simulink model "SIM_DNNs"  (R2024a)
settings: Solver=VariableStepAuto  StartTime=0.0  StopTime=xs.sim.Tf2  FixedStep=1e-4  RelTol=1e-3
values from neighbouring files (symbols this model uses):
  eval_net_func1 = Simulink.Parameter    [InitMain.m]    (also in InitMain_original.m)
  eval_net_func2 = Simulink.Parameter    [InitMain.m]    (also in InitMain_original.m)
  mins_max1 = Simulink.Parameter    [InitMain.m]    (also in InitMain_original.m)
  mins_max2 = Simulink.Parameter    [InitMain.m]    (also in InitMain_original.m)
  parsDNN1 = Simulink.Parameter    [InitMain.m]    (also in InitMain_original.m)
  parsDNN2 = Simulink.Parameter    [InitMain.m]    (also in InitMain_original.m)
  use_net1 = Simulink.Parameter    [InitMain.m]    (also in InitMain_original.m)
  use_net2 = Simulink.Parameter    [InitMain.m]    (also in InitMain_original.m)
  xmpc1 = xs.MPC1    [InitMPCs.m]
  xmpc2 = xs.MPC2    [InitMPCs.m]
  xproj1 = xs.Proj1    [InitMPCs.m]
  xs = xs_us(1:4)    [MPC1_f.m]    (also in MPC2_f.m = xs_us(1:3))
undefined symbols (not defined in the file or in its folder): Lf, Rf, xsat2
libraries: spsThreePhaseSeriesRLCBranchLib x4, spsThreePhaseVIMeasurementLib x3, spsTriangleGeneratorLib x2, spsDCVoltageSourceLib x1, spsThreePhaseBreakerLib x1, spsThreePhaseSourceLib x1, spsTwoLevelConverterLib x1, sps_lib x1
settings Model: Creator=iaaco  LastModifiedBy=fabus
settings SolverCC: ShapePreserveControl=EnableAll
settings OptimizationCC: DefaultParameterBehavior=Inlined  EnhancedBackFolding=on  PassReuseOutputArgsAs=Individual arguments  ZeroExternalMemoryAtStartup=off  ZeroInternalMemoryAtStartup=off  OptimizeBlockOrder=speed  DifferentSizesBufferReuse=on  OptimizationCustomize=off  EfficientTunableParamExpr=on
settings DebuggingCC: ParameterTunabilityLossMsg=error
settings RTWCC: Description=Embedded Coder  SystemTargetFile=ert.tlc  TemplateMakefile=ert_default_tmf
settings CodeAppCC: ForceParamTrailComments=on  IgnoreCustomStorageClasses=off  OperatorAnnotations=on  SimulinkDataObjDesc=on  SFDataObjDesc=on  InsertBlockDesc=on
settings ERTTargetCC: TargetLangStandard=C99 (ISO)  GenerateSampleERTMain=on  InlinedParameterPlacement=NonHierarchical  ERTCustomFileTemplate=example_file_process.tlc

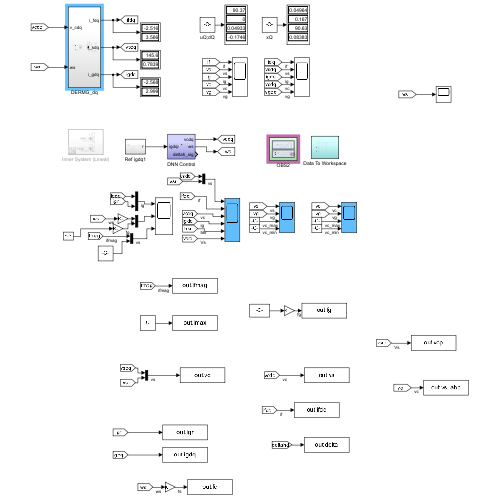
[thumbnail: Simulink's stored preview of the top-level diagram]
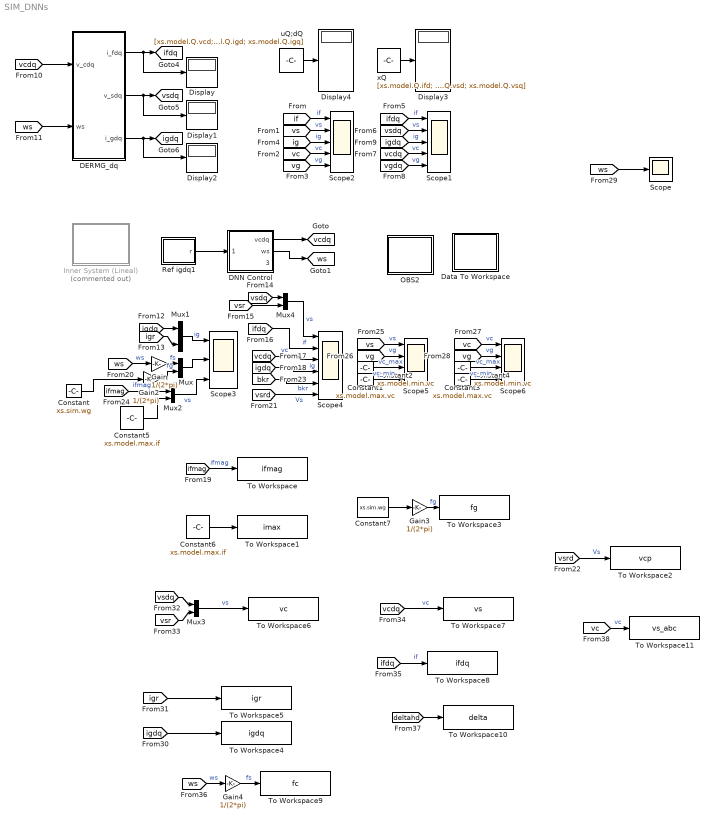
== system SIM_DNNs ==
  Constant : Constant  Value=xs.sim.wg
  Constant1 : Constant  Value=xs.model.max.vc
  Constant2 : Constant  Value=xs.model.min.vc
  Constant3 : Constant  Value=xs.model.max.vc
  Constant4 : Constant  Value=xs.model.min.vc
  Constant5 : Constant  Value=xs.model.max.if
  Constant6 : Constant  Value=xs.model.max.if
  Constant7 : Constant  Value=xs.sim.wg
  DERMG_dq : Subsystem
  DNN Control : Subsystem
  Data To Workspace : Subsystem
  Display{,1..4} (5 alike) : Display
  Gain{,2..4} (4 alike) : Gain  Gain=1/(2*pi)
  Inner System (Lineal) : Subsystem  Commented=on
  Mux{,1..4} (5 alike) : Mux  Inputs=2
  OBS2 : Subsystem
  Ref igdq1 : Subsystem
  Scope : Scope
  Scope1 : Scope  NumInputPorts=5
  Scope2 : Scope  NumInputPorts=5
  Scope3 : Scope  NumInputPorts=3
  Scope4 : Scope  NumInputPorts=6
  Scope5 : Scope  NumInputPorts=4
  Scope6 : Scope  NumInputPorts=4
  To Workspace : ToWorkspace  VariableName=ifmag  SampleTime=-1
  To Workspace1 : ToWorkspace  VariableName=imax  SampleTime=-1
  To Workspace10 : ToWorkspace  VariableName=delta  SaveFormat=Timeseries  SampleTime=-1
  To Workspace11 : ToWorkspace  VariableName=vs_abc  SaveFormat=Timeseries  SampleTime=-1
  To Workspace2 : ToWorkspace  VariableName=vcp  SaveFormat=Timeseries  SampleTime=-1
  To Workspace3 : ToWorkspace  VariableName=fg  SampleTime=-1
  To Workspace4 : ToWorkspace  VariableName=igdq  SaveFormat=Timeseries  SampleTime=-1
  To Workspace5 : ToWorkspace  VariableName=igr  SaveFormat=Timeseries  SampleTime=-1
  To Workspace6 : ToWorkspace  VariableName=vc  SaveFormat=Timeseries  SampleTime=-1
  To Workspace7 : ToWorkspace  VariableName=vs  SaveFormat=Timeseries  SampleTime=-1
  To Workspace8 : ToWorkspace  VariableName=ifdq  SaveFormat=Timeseries  SampleTime=-1
  To Workspace9 : ToWorkspace  VariableName=fc  SaveFormat=Timeseries  SampleTime=-1
  uQ;dQ : Constant  Value=[xs.model.Q.vcd; xs.model.Q.vcq; xs.model.Q.igd; xs.model.Q.igq]
  xQ : Constant  Value=[xs.model.Q.ifd; xs.model.Q.ifq; xs.model.Q.vsd; xs.model.Q.vsq]
  tag scope: ifdq=global, igdq=global, vcdq=global, vsdq=global, ws=global
  wires:
  [vcdq] -> Scope1/4  "vc"
  [ifdq] -> Scope1/1  "if"
  [vgdq] -> Scope1/5  "vg"
  [igdq] -> Scope1/3  "ig"
  [vsdq] -> Scope1/2  "vs"
  [vcdq] -> DERMG_dq/1(v_cdq)
  [ws] -> DERMG_dq/2(ws)
  DERMG_dq/1(i_fdq) -> Display/1, [ifdq]
  DERMG_dq/2(v_sdq) -> Display1/1, [vsdq]
  DERMG_dq/3(i_gdq) -> Display2/1, [igdq]
  xQ/1 -> Display3/1
  uQ;dQ/1 -> Display4/1
  Ref igdq1/1(r) -> DNN Control/1(igdqr)
  DNN Control/1(vcdq) -> [vcdq]
  DNN Control/2(ws) -> [ws]
  [ig] -> Scope2/3  "ig"
  [vs] -> Scope2/2  "vs"
  [vg] -> Scope2/5  "vg"
  [if] -> Scope2/1  "if"
  [vc] -> Scope2/4  "vc"
  Constant4/1 -> Scope6/4  "vc_min"
  Gain2/1 -> Mux/2  "fg"
  Constant3/1 -> Scope6/3  "vc_max"
  [vc] -> Scope6/1  "vc"
  [vg] -> Scope5/2  "vg"
  [igr] -> Mux1/2
  Gain/1 -> Mux/1  "fs"
  Mux/1 -> Scope3/2
  [vcdq] -> Scope4/3  "vc"
  [bkr] -> Scope4/5  "bkr"
  [vg] -> Scope6/2  "vg"
  [vs] -> Scope5/1  "vs"
  [igdq] -> Mux1/1
  Constant1/1 -> Scope5/3  "vc_max"
  Constant/1 -> Gain2/1
  Constant2/1 -> Scope5/4  "vc_min"
  [igdq] -> Scope4/4  "ig"
  [vsdq] -> Mux4/1
  Mux4/1 -> Scope4/1  "vs"
  [vsrd] -> Scope4/6  "Vs"
  [ws] -> Gain/1  "ws"
  [vsr] -> Mux4/2
  Mux1/1 -> Scope3/1  "ig"
  [ws] -> Scope/1
  [ifdq] -> Scope4/2  "if"
  Constant5/1 -> Mux2/2
  [ifmag] -> Mux2/1  "ifmag"
  Mux2/1 -> Scope3/3  "vs"
  [ifmag] -> To Workspace/1  "ifmag"
  Constant6/1 -> To Workspace1/1
  Constant7/1 -> Gain3/1
  Gain3/1 -> To Workspace3/1  "fg"
  [igdq] -> To Workspace4/1
  [igr] -> To Workspace5/1
  Mux3/1 -> To Workspace6/1  "vs"
  [vsr] -> Mux3/2
  [vsdq] -> Mux3/1
  [vcdq] -> To Workspace7/1  "vc"
  [ifdq] -> To Workspace8/1  "if"
  [ws] -> Gain4/1  "ws"
  Gain4/1 -> To Workspace9/1  "fs"
  [vsrd] -> To Workspace2/1  "Vs"
  [deltahd] -> To Workspace10/1
  [vc] -> To Workspace11/1  "vc"

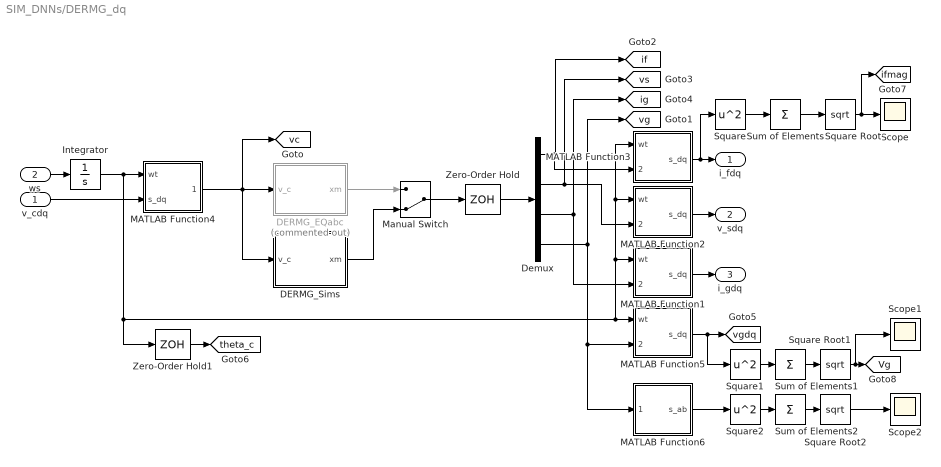
== system SIM_DNNs/DERMG_dq ==
  v_cdq : Inport
  ws : Inport  Port=2
  DERMG_EQabc : Subsystem  Commented=on
  DERMG_Sims : Subsystem
  Demux : Demux
  Integrator : Integrator  WrapState=on
  MATLAB Function1 : MATLAB Function  TreatAsAtomicUnit=on
  MATLAB Function2 : MATLAB Function  TreatAsAtomicUnit=on
  MATLAB Function3 : MATLAB Function  TreatAsAtomicUnit=on
  MATLAB Function4 : MATLAB Function  TreatAsAtomicUnit=on
  MATLAB Function5 : MATLAB Function  TreatAsAtomicUnit=on
  MATLAB Function6 : MATLAB Function  TreatAsAtomicUnit=on
  Manual Switch : ManualSwitch  CurrentSetting=0
  Scope : Scope
  Scope1 : Scope
  Scope2 : Scope
  Square : Math  Operator=square
  Square Root : Sqrt
  Square Root1 : Sqrt
  Square Root2 : Sqrt
  Square1 : Math  Operator=square
  Square2 : Math  Operator=square
  Sum of Elements : Sum  Inputs=+
  Sum of Elements1 : Sum  Inputs=+
  Sum of Elements2 : Sum  Inputs=+
  Zero-Order Hold : ZeroOrderHold  SampleTime=xs.model.Ts
  Zero-Order Hold1 : ZeroOrderHold  SampleTime=xs.model.Ts
  i_fdq : Outport
  v_sdq : Outport  Port=2
  i_gdq : Outport  Port=3
  tag scope: Vg=global, if=global, ifmag=global, ig=global, theta_c=global, vc=global, vg=global, vgdq=global, vs=global
  wires:
  MATLAB Function3/1(s_dq) -> Square/1, i_fdq/1
  MATLAB Function2/1(s_dq) -> v_sdq/1
  MATLAB Function1/1(s_dq) -> i_gdq/1
  ws/1 -> Integrator/1
  Square/1 -> Sum of Elements/1
  Sum of Elements/1 -> Square Root/1
  Integrator/1 -> MATLAB Function5/1(wt), MATLAB Function1/1(wt), MATLAB Function3/1(wt), MATLAB Function2/1(wt), Zero-Order Hold1/1, MATLAB Function4/1(wt)
  Demux/1 -> MATLAB Function3/2(s_abc), [if]
  Demux/2 -> MATLAB Function2/2(s_abc), [vs]
  Demux/3 -> MATLAB Function1/2(s_abc), [ig]
  Demux/4 -> MATLAB Function6/1(s_abc), MATLAB Function5/2(s_abc), [vg]
  Square Root/1 -> [ifmag], Scope/1
  Zero-Order Hold/1 -> Demux/1
  Zero-Order Hold1/1 -> [theta_c]
  MATLAB Function4/1(s_abc) -> [vc], DERMG_Sims/1(v_c), DERMG_EQabc/1(v_c)
  Manual Switch/1 -> Zero-Order Hold/1
  DERMG_EQabc/1(xm) -> Manual Switch/1
  DERMG_Sims/1(xm) -> Manual Switch/2
  Sum of Elements1/1 -> Square Root1/1
  MATLAB Function5/1(s_dq) -> Square1/1, [vgdq]
  Square1/1 -> Sum of Elements1/1
  Square Root1/1 -> Scope1/1, [Vg]
  Square Root2/1 -> Scope2/1
  Square2/1 -> Sum of Elements2/1
  Sum of Elements2/1 -> Square Root2/1
  MATLAB Function6/1(s_ab) -> Square2/1
  v_cdq/1 -> MATLAB Function4/2(s_dq)

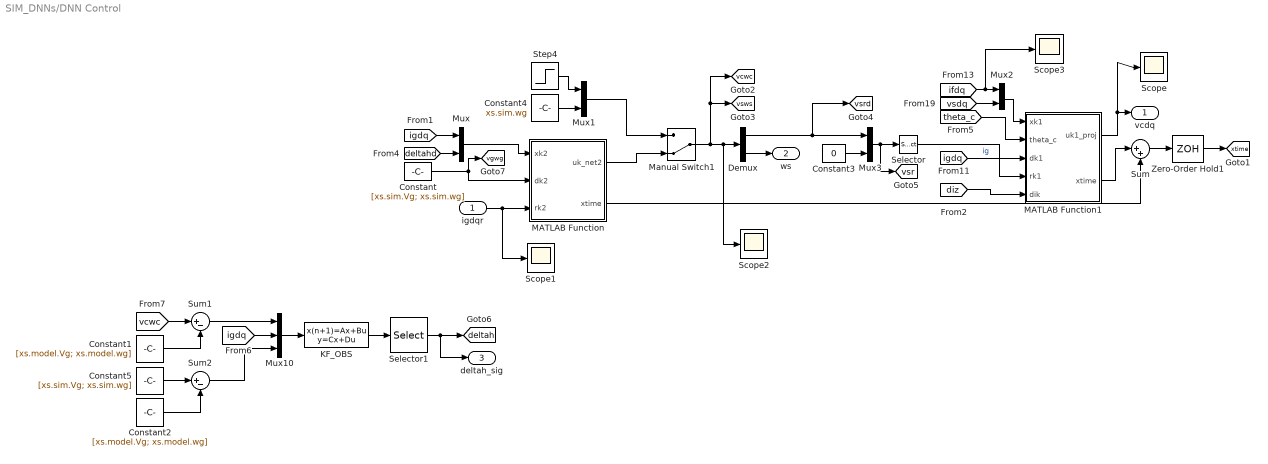
== system SIM_DNNs/DNN Control ==
  igdqr : Inport
  Constant : Constant  Value=[xs.sim.Vg; xs.sim.wg]
  Constant1 : Constant  Value=[xs.model.Vg; xs.model.wg]
  Constant2 : Constant  Value=[xs.model.Vg; xs.model.wg]
  Constant3 : Constant  Value=0
  Constant4 : Constant  Value=xs.sim.wg
  Constant5 : Constant  Value=[xs.sim.Vg; xs.sim.wg]
  Demux : Demux  Outputs=2
  KF_OBS : DiscreteStateSpace  A=xs.model.Ad2-xs.OBS2.L*xs.model.C2s  B=[xs.model.Bd2 ,xs.OBS2.L,xs.model.Bod2]  C=eye(3)  D=zeros(3,6)  InitialCondition=zeros(3,1)  SampleTime=xs.model.Ts
  MATLAB Function : MATLAB Function  TreatAsAtomicUnit=on  SystemSampleTime=xs.model.Ts
  MATLAB Function1 : MATLAB Function  TreatAsAtomicUnit=on  SystemSampleTime=xs.model.Ts
  Manual Switch1 : ManualSwitch  CurrentSetting=0
  Mux{,1..3} (4 alike) : Mux  Inputs=2
  Mux10 : Mux  Inputs=3
  Scope{,1..3} (4 alike) : Scope
  Selector : Selector  InputPortWidth=2  IndexOptions=Index vector (dialog)  Indices=[1]  OutputSizes=1
  Selector1 : Selector  InputPortWidth=3  IndexOptions=Index vector (dialog)  Indices=[3]  OutputSizes=1
  Step4 : Step  Time=xs.sim.vsdr.Tstep  Before=90  After=xs.sim.vsdr.XF  SampleTime=0
  Sum : Sum  Inputs=|++
  Sum1 : Sum  Inputs=|+-
  Sum2 : Sum  Inputs=|+-
  Zero-Order Hold1 : ZeroOrderHold  SampleTime=xs.model.Ts
  vcdq : Outport
  ws : Outport  Port=2
  deltah_sig : Outport  Port=3
  tag scope: deltah=global, vcwc=global, vgwg=global, vsr=global, vsrd=global, vsws=global, xtime=global
  wires:
  Manual Switch1/1 -> [vcwc], [vsws], Scope2/1, Demux/1
  Mux1/1 -> Manual Switch1/1
  [deltahd] -> Mux/2
  Constant/1 -> [vgwg], MATLAB Function/2(dk2)
  [igdq] -> Mux/1
  Mux/1 -> MATLAB Function/1(xk2)
  igdqr/1 -> Scope1/1, MATLAB Function/3(rk2)
  MATLAB Function/1(uk_net2) -> Manual Switch1/2
  [ifdq] -> Scope3/1, Mux2/1
  Constant3/1 -> Mux3/2
  [vsdq] -> Mux2/2
  Mux3/1 -> Selector/1, [vsr]
  Demux/1 -> Mux3/1, [vsrd]
  Mux2/1 -> MATLAB Function1/1(xk1)
  Demux/2 -> ws/1
  [theta_c] -> MATLAB Function1/2(theta_c)
  Constant4/1 -> Mux1/2
  Step4/1 -> Mux1/1
  MATLAB Function1/1(uk1_proj) -> Scope/1, vcdq/1
  MATLAB Function1/2(xtime) -> Sum/1
  MATLAB Function/2(xtime) -> Sum/2
  Sum/1 -> Zero-Order Hold1/1
  Zero-Order Hold1/1 -> [xtime]
  Selector/1 -> MATLAB Function1/4(rk1)
  [igdq] -> MATLAB Function1/3(dk1)  "ig"
  [diz] -> MATLAB Function1/5(dik)
  Mux10/1 -> KF_OBS/1
  Sum1/1 -> Mux10/1
  [vcwc] -> Sum1/1
  [igdq] -> Mux10/2
  Constant5/1 -> Sum2/1
  KF_OBS/1 -> Selector1/1
  Constant1/1 -> Sum1/2
  Sum2/1 -> Mux10/3
  Selector1/1 -> deltah_sig/1, [deltah]
  Constant2/1 -> Sum2/2

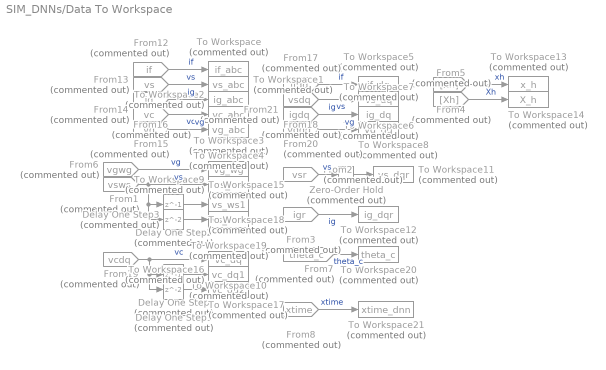
== system SIM_DNNs/Data To Workspace ==
  Delay One Step : Delay  Commented=on  DelayLength=1  SampleTime=xs.model.Ts
  Delay One Step1 : Delay  Commented=on  SampleTime=xs.model.Ts
  Delay One Step2 : Delay  Commented=on  DelayLength=1  SampleTime=xs.model.Ts
  Delay One Step3 : Delay  Commented=on  SampleTime=xs.model.Ts
  From1 : From  Commented=on  GotoTag=vsws  TagVisibility=global
  From12 : From  Commented=on  GotoTag=if  TagVisibility=global
  From13 : From  Commented=on  GotoTag=vs  TagVisibility=global
  From14 : From  Commented=on  GotoTag=vc  TagVisibility=global
  From15 : From  Commented=on  GotoTag=vg  TagVisibility=global
  From16 : From  Commented=on  GotoTag=ig  TagVisibility=global
  From17 : From  Commented=on  GotoTag=ifdq  TagVisibility=global
  From18 : From  Commented=on  GotoTag=vsdq  TagVisibility=global
  From19 : From  Commented=on  GotoTag=vcdq  TagVisibility=global
  From2 : From  Commented=on  GotoTag=vsr  TagVisibility=global
  From20 : From  Commented=on  GotoTag=vgdq  TagVisibility=global
  From21 : From  Commented=on  GotoTag=igdq  TagVisibility=global
  From3 : From  Commented=on  GotoTag=igr  TagVisibility=global
  From4 : From  Commented=on  GotoTag=xh
  From5 : From  Commented=on  GotoTag=Xh
  From6 : From  Commented=on  GotoTag=vgwg  TagVisibility=global
  From7 : From  Commented=on  GotoTag=theta_c  TagVisibility=global
  From8 : From  Commented=on  GotoTag=xtime  TagVisibility=global
  To Workspace : ToWorkspace  Commented=on  VariableName=if_abc  SaveFormat=Structure With Time  SampleTime=xs.model.Ts
  To Workspace1 : ToWorkspace  Commented=on  VariableName=vs_abc  SaveFormat=Structure With Time  SampleTime=xs.model.Ts
  To Workspace10 : ToWorkspace  Commented=on  VariableName=vc_dq  SaveFormat=Structure With Time  SampleTime=xs.model.Ts
  To Workspace11 : ToWorkspace  Commented=on  VariableName=vs_dqr  SaveFormat=Structure With Time  SampleTime=xs.model.Ts
  To Workspace12 : ToWorkspace  Commented=on  VariableName=ig_dqr  SaveFormat=Structure With Time  SampleTime=xs.model.Ts
  To Workspace13 : ToWorkspace  Commented=on  VariableName=x_h  SaveFormat=Structure With Time  SampleTime=xs.model.Ts
  To Workspace14 : ToWorkspace  Commented=on  VariableName=X_h  SaveFormat=Structure With Time  SampleTime=xs.model.Ts
  To Workspace15 : ToWorkspace  Commented=on  VariableName=vg_wg  SaveFormat=Structure With Time  SampleTime=xs.model.Ts
  To Workspace16 : ToWorkspace  Commented=on  VariableName=vc_dq1  SaveFormat=Structure With Time  SampleTime=xs.model.Ts
  To Workspace17 : ToWorkspace  Commented=on  VariableName=vc_dq2  SaveFormat=Structure With Time  SampleTime=xs.model.Ts
  To Workspace18 : ToWorkspace  Commented=on  VariableName=vs_ws1  SaveFormat=Structure With Time  SampleTime=xs.model.Ts
  To Workspace19 : ToWorkspace  Commented=on  VariableName=vs_ws2  SaveFormat=Structure With Time  SampleTime=xs.model.Ts
  To Workspace2 : ToWorkspace  Commented=on  VariableName=ig_abc  SaveFormat=Structure With Time  SampleTime=xs.model.Ts
  To Workspace20 : ToWorkspace  Commented=on  VariableName=theta_c  SaveFormat=Structure With Time  SampleTime=xs.model.Ts
  To Workspace21 : ToWorkspace  Commented=on  VariableName=xtime_dnn  SaveFormat=Structure With Time  SampleTime=xs.model.Ts
  To Workspace3 : ToWorkspace  Commented=on  VariableName=vc_abc  SaveFormat=Structure With Time  SampleTime=xs.model.Ts
  To Workspace4 : ToWorkspace  Commented=on  VariableName=vg_abc  SaveFormat=Structure With Time  SampleTime=xs.model.Ts
  To Workspace5 : ToWorkspace  Commented=on  VariableName=if_dq  SaveFormat=Structure With Time  SampleTime=xs.model.Ts
  To Workspace6 : ToWorkspace  Commented=on  VariableName=vs_dq  SaveFormat=Structure With Time  SampleTime=xs.model.Ts
  To Workspace7 : ToWorkspace  Commented=on  VariableName=ig_dq  SaveFormat=Structure With Time  SampleTime=xs.model.Ts
  To Workspace8 : ToWorkspace  Commented=on  VariableName=vg_dq  SaveFormat=Structure With Time  SampleTime=xs.model.Ts
  To Workspace9 : ToWorkspace  Commented=on  VariableName=vs_ws  SaveFormat=Structure With Time  SampleTime=xs.model.Ts
  Zero-Order Hold : ZeroOrderHold  Commented=on  SampleTime=xs.model.Ts
  wires:
  From12/1 -> To Workspace/1  "if"
  From13/1 -> To Workspace1/1  "vs"
  From16/1 -> To Workspace2/1  "ig"
  From14/1 -> To Workspace3/1  "vc"
  From15/1 -> To Workspace4/1  "vg"
  From17/1 -> To Workspace5/1  "if"
  From18/1 -> To Workspace6/1  "vs"
  From21/1 -> To Workspace7/1  "ig"
  From20/1 -> To Workspace8/1  "vg"
  From1/1 -> Delay One Step3/1, Delay One Step2/1, To Workspace9/1  "vs"
  From19/1 -> Delay One Step1/1, Delay One Step/1, To Workspace10/1  "vc"
  From3/1 -> To Workspace12/1  "ig"
  Zero-Order Hold/1 -> To Workspace11/1
  From4/1 -> To Workspace13/1  "xh"
  From5/1 -> To Workspace14/1  "Xh"
  From6/1 -> To Workspace15/1  "vg"
  From2/1 -> Zero-Order Hold/1  "vs"
  Delay One Step/1 -> To Workspace16/1
  Delay One Step1/1 -> To Workspace17/1
  Delay One Step2/1 -> To Workspace18/1
  Delay One Step3/1 -> To Workspace19/1
  From7/1 -> To Workspace20/1  "theta_c"
  From8/1 -> To Workspace21/1  "xtime"

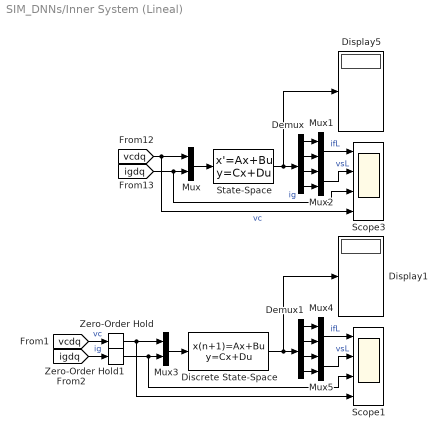
== system SIM_DNNs/Inner System (Lineal) ==
  Demux : Demux
  Demux1 : Demux
  Discrete State-Space : DiscreteStateSpace  A=xs.model.Ad1  B=[xs.model.Bd1,xs.model.Bod1]  C=eye(4)  D=zeros(4)  InitialCondition=[xs.model.Q.ifd ; xs.model.Q.ifq ; xs.model.Q.vsd ; xs.model.Q.vsq]  SampleTime=xs.model.Ts
  Display1 : Display
  Display5 : Display
  Mux{,1..5} (6 alike) : Mux  Inputs=2
  Scope1 : Scope  NumInputPorts=4
  Scope3 : Scope  NumInputPorts=4
  State-Space : StateSpace  A=xs.model.A1  B=[xs.model.B1,xs.model.Bo1]  C=eye(4)  D=zeros(4)  InitialCondition=[xs.model.Q.ifd ; xs.model.Q.ifq ; xs.model.Q.vsd ; xs.model.Q.vsq]
  Zero-Order Hold : ZeroOrderHold  SampleTime=xs.model.Ts
  Zero-Order Hold1 : ZeroOrderHold  SampleTime=xs.model.Ts
  wires:
  Mux/1 -> State-Space/1
  Demux/1 -> Mux1/1
  Demux/2 -> Mux1/2
  State-Space/1 -> Display5/1, Demux/1
  [vcdq] -> Scope3/4, Mux/1  "vc"
  [igdq] -> Scope3/3, Mux/2  "ig"
  Mux2/1 -> Scope3/2  "vsL"
  Mux1/1 -> Scope3/1  "ifL"
  Demux/3 -> Mux2/1
  Demux/4 -> Mux2/2
  Demux1/4 -> Mux5/2
  [vcdq] -> Zero-Order Hold/1  "vc"
  Mux5/1 -> Scope1/2  "vsL"
  Demux1/2 -> Mux4/2
  Mux3/1 -> Discrete State-Space/1
  [igdq] -> Zero-Order Hold1/1  "ig"
  Demux1/1 -> Mux4/1
  Mux4/1 -> Scope1/1  "ifL"
  Demux1/3 -> Mux5/1
  Discrete State-Space/1 -> Display1/1, Demux1/1
  Zero-Order Hold/1 -> Scope1/4, Mux3/1
  Zero-Order Hold1/1 -> Scope1/3, Mux3/2

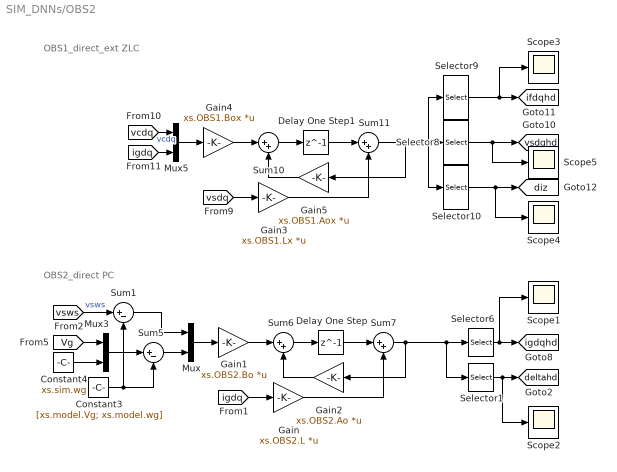
== system SIM_DNNs/OBS2 ==
  note: OBS1_direct_ext ZLC
  note: OBS2_direct PC
  Constant3 : Constant  Value=[xs.model.Vg; xs.model.wg]
  Constant4 : Constant  Value=xs.sim.wg
  Delay One Step : Delay  DelayLength=1  InitialCondition=zeros(3,1)  SampleTime=xs.model.Ts
  Delay One Step1 : Delay  DelayLength=1  InitialCondition=zeros(6,1)  SampleTime=xs.model.Ts
  Gain : Gain  Gain=xs.OBS2.L  Multiplication=Matrix(K*u)
  Gain1 : Gain  Gain=xs.OBS2.Bo  Multiplication=Matrix(K*u)
  Gain2 : Gain  Gain=xs.OBS2.Ao  Multiplication=Matrix(K*u)
  Gain3 : Gain  Gain=xs.OBS1.Lx  Multiplication=Matrix(K*u)
  Gain4 : Gain  Gain=xs.OBS1.Box  Multiplication=Matrix(K*u)
  Gain5 : Gain  Gain=xs.OBS1.Aox  Multiplication=Matrix(K*u)
  Mux : Mux  Inputs=2
  Mux3 : Mux  Inputs=2
  Mux5 : Mux  Inputs=2
  Scope{1..5} (5 alike) : Scope
  Selector1 : Selector  InputPortWidth=3  IndexOptions=Index vector (dialog)  Indices=[3]  OutputSizes=1
  Selector10 : Selector  InputPortWidth=6  IndexOptions=Index vector (dialog)  Indices=[5 6]  OutputSizes=1
  Selector6 : Selector  InputPortWidth=3  IndexOptions=Index vector (dialog)  Indices=[1 2]  OutputSizes=1
  Selector8 : Selector  InputPortWidth=6  IndexOptions=Index vector (dialog)  Indices=[3 4]  OutputSizes=1
  Selector9 : Selector  InputPortWidth=6  IndexOptions=Index vector (dialog)  Indices=[1 2]  OutputSizes=1
  Sum1 : Sum  Inputs=|+-
  Sum{6..7,10..11} (4 alike) : Sum  Inputs=|++
  Sum5 : Sum  Inputs=|+-
  tag scope: deltahd=global, diz=global, ifdqhd=global, igdqhd=global, vsdqhd=global
  wires:
  Sum11/1 -> Selector9/1, Selector10/1, Selector8/1, Gain5/1
  Gain4/1 -> Sum10/1
  [vsdq] -> Gain3/1
  [vsws] -> Sum1/1  "vsws"
  [vcdq] -> Mux5/1  "vcdq"
  Gain1/1 -> Sum6/1
  Gain2/1 -> Sum6/2
  [igdq] -> Gain/1
  Mux/1 -> Gain1/1
  Sum7/1 -> Selector1/1, Selector6/1, Gain2/1
  [igdq] -> Mux5/2
  Selector6/1 -> Scope1/1, [igdqhd]
  Sum6/1 -> Delay One Step/1
  Sum1/1 -> Mux/1
  Sum5/1 -> Mux/2
  Constant4/1 -> Mux3/2
  Mux3/1 -> Sum5/1
  Selector1/1 -> Scope2/1, [deltahd]
  [Vg] -> Mux3/1
  Constant3/1 -> Sum5/2, Sum1/2
  Selector9/1 -> [ifdqhd], Scope3/1
  Gain3/1 -> Sum11/2
  Delay One Step1/1 -> Sum11/1
  Selector8/1 -> Scope5/1, [vsdqhd]
  Mux5/1 -> Gain4/1
  Selector10/1 -> Scope4/1, [diz]
  Delay One Step/1 -> Sum7/1
  Gain/1 -> Sum7/2
  Gain5/1 -> Sum10/2
  Sum10/1 -> Delay One Step1/1

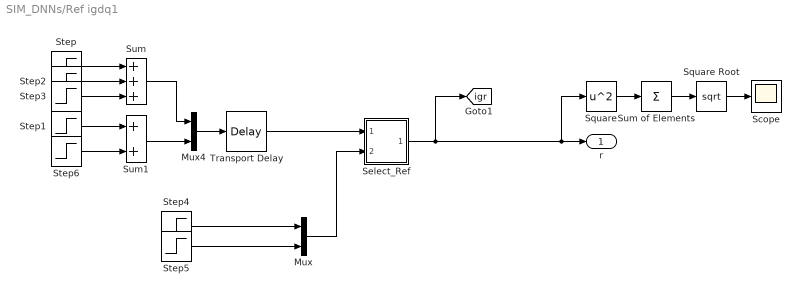
== system SIM_DNNs/Ref igdq1 ==
  Mux : Mux  Inputs=2
  Mux4 : Mux  Inputs=2
  Scope : Scope
  Select_Ref : Subsystem
  Square : Math  Operator=square
  Square Root : Sqrt
  Step : Step  Time=xs.sim.Tf2*0.25  Before=3  After=7  SampleTime=0
  Step1 : Step  Time=xs.sim.Tf2*0.5  After=-7  SampleTime=0
  Step2 : Step  Time=xs.sim.Tf2*0.5  After=-7  SampleTime=0
  Step3 : Step  Time=xs.sim.Tf2*0.75  After=-3  SampleTime=0
  Step4 : Step  Time=xs.sim.igdr.Tstep  Before=xs.sim.igdr.X0  After=xs.sim.igdr.XF  SampleTime=0
  Step5 : Step  Time=xs.sim.igqr.Tstep  Before=xs.sim.igqr.X0  After=xs.sim.igqr.XF  SampleTime=0
  Step6 : Step  Time=xs.sim.Tf2*0.75  After=10  SampleTime=0
  Sum : Sum  Inputs=+++
  Sum of Elements : Sum  Inputs=+
  Sum1 : Sum
  Transport Delay : TransportDelay  DelayTime=0.1  BufferSize=23000
  r : Outport
  tag scope: igr=global
  wires:
  Step4/1 -> Mux/1
  Step5/1 -> Mux/2
  Square Root/1 -> Scope/1
  Square/1 -> Sum of Elements/1
  Select_Ref/1(r2k) -> r/1, Square/1, [igr]
  Sum of Elements/1 -> Square Root/1
  Mux/1 -> Select_Ref/2(In2)
  Transport Delay/1 -> Select_Ref/1(In1)
  Step6/1 -> Sum1/2
  Step3/1 -> Sum/3
  Mux4/1 -> Transport Delay/1
  Step2/1 -> Sum/2
  Step/1 -> Sum/1
  Step1/1 -> Sum1/1
  Sum1/1 -> Mux4/2
  Sum/1 -> Mux4/1

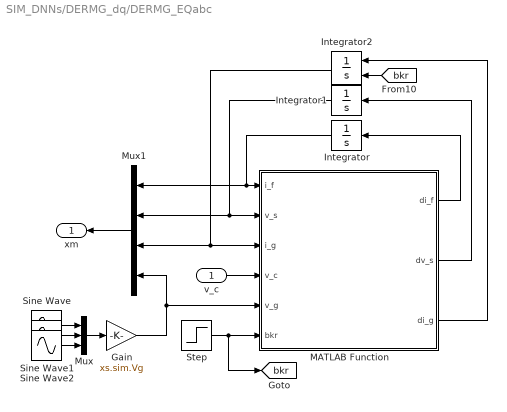
== system SIM_DNNs/DERMG_dq/DERMG_EQabc ==
  v_c : Inport
  Gain : Gain  Gain=xs.sim.Vg
  Integrator : Integrator  InitialCondition=xs.sim.X0abc.if*0
  Integrator1 : Integrator  InitialCondition=xs.sim.X0abc.vs*0
  Integrator2 : Integrator  ExternalReset=falling  InitialCondition=xs.sim.X0abc.ig*0
  MATLAB Function : MATLAB Function  TreatAsAtomicUnit=on
  Mux : Mux  Inputs=3
  Mux1 : Mux
  Sine Wave : Sin  Frequency=xs.sim.wg  Phase=0 + pi/2- xs.sim.thetag0  SampleTime=0
  Sine Wave1 : Sin  Frequency=xs.sim.wg  Phase=-2*pi/3 + pi/2 - xs.sim.thetag0  SampleTime=0
  Sine Wave2 : Sin  Frequency=xs.sim.wg  Phase=-4*pi/3 + pi/2 - xs.sim.thetag0  SampleTime=0
  Step : Step  Time=xs.sim.bkr.Tstep  Before=xs.sim.bkr.X0  After=xs.sim.bkr.XF  SampleTime=0
  xm : Outport
  tag scope: bkr=global
  wires:
  Integrator/1 -> MATLAB Function/1(i_f), Mux1/1
  MATLAB Function/3(di_g) -> Integrator2/1
  Integrator2/1 -> Mux1/3, MATLAB Function/3(i_g)
  MATLAB Function/2(dv_s) -> Integrator1/1
  Integrator1/1 -> Mux1/2, MATLAB Function/2(v_s)
  v_c/1 -> MATLAB Function/4(v_c)
  MATLAB Function/1(di_f) -> Integrator/1
  Sine Wave/1 -> Mux/1
  Mux/1 -> Gain/1
  Sine Wave2/1 -> Mux/3
  Sine Wave1/1 -> Mux/2
  Gain/1 -> MATLAB Function/5(v_g), Mux1/4
  Mux1/1 -> xm/1
  Step/1 -> [bkr], MATLAB Function/6(bkr)
  [bkr] -> Integrator2/2

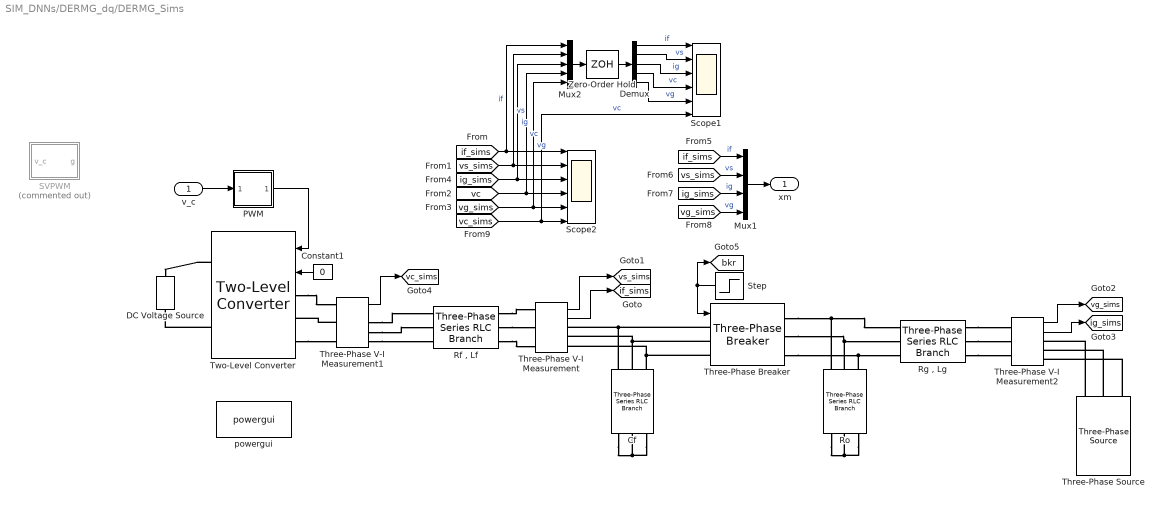
== system SIM_DNNs/DERMG_dq/DERMG_Sims ==
  v_c : Inport
  Cf : spsThreePhaseSeriesRLCBranchLib/Three-Phase Series RLC Branch  LConnTagsString=A|B|C  RConnTagsString=A|B|C  BranchType=C  Resistance=Rf  Inductance=Lf  Capacitance=xs.sim.Cf  Measurements=None
  Constant1 : Constant  Value=0
  DC Voltage Source : spsDCVoltageSourceLib/DC Voltage Source  Amplitude=xs.sim.vdc  Measurements=None
  Demux : Demux  Outputs=5
  Mux1 : Mux
  Mux2 : Mux  Inputs=5
  PWM : Subsystem
  "Rf , Lf" : spsThreePhaseSeriesRLCBranchLib/Three-Phase Series RLC Branch  LConnTagsString=A|B|C  RConnTagsString=A|B|C  BranchType=RL  Resistance=xs.sim.Rf  Inductance=xs.sim.Lf  Capacitance=0  Measurements=None
  "Rg , Lg" : spsThreePhaseSeriesRLCBranchLib/Three-Phase Series RLC Branch  LConnTagsString=A|B|C  RConnTagsString=A|B|C  BranchType=RL  Resistance=xs.sim.Rg  Inductance=xs.sim.Lg  Capacitance=0  Measurements=None
  Ro : spsThreePhaseSeriesRLCBranchLib/Three-Phase Series RLC Branch  LConnTagsString=A|B|C  RConnTagsString=A|B|C  BranchType=R  Resistance=xs.sim.Ro  Inductance=Lf  Capacitance=xs.sim.Cf  Measurements=None
  SVPWM : Subsystem  Commented=on
  Scope1 : Scope  NumInputPorts=6
  Scope2 : Scope  NumInputPorts=6
  Step : Step  Time=xs.sim.bkr.Tstep  Before=xs.sim.bkr.X0  After=xs.sim.bkr.XF  SampleTime=0
  Three-Phase V-I Measurement : spsThreePhaseVIMeasurementLib/Three-Phase V-I Measurement  VoltageMeasurement=phase-to-ground  SetLabelV=off  LabelV=Vabc  Vpu=off  VpuLL=off  CurrentMeasurement=yes  SetLabelI=off  LabelI=Iabc  Ipu=off  Pbase=100e6  Vbase=500e3  OutputType=Complex  PhasorSimulation=off  PSBequivalent=0
  Three-Phase V-I Measurement1 : spsThreePhaseVIMeasurementLib/Three-Phase V-I Measurement  VoltageMeasurement=phase-to-ground  SetLabelV=off  LabelV=Vabc  Vpu=off  VpuLL=off  CurrentMeasurement=yes  SetLabelI=off  LabelI=Iabc  Ipu=off  Pbase=100e6  Vbase=500e3  OutputType=Complex  PhasorSimulation=off  PSBequivalent=0
  Three-Phase V-I Measurement2 : spsThreePhaseVIMeasurementLib/Three-Phase V-I Measurement  VoltageMeasurement=phase-to-ground  SetLabelV=off  LabelV=Vabc  Vpu=off  VpuLL=off  CurrentMeasurement=yes  SetLabelI=off  LabelI=Iabc  Ipu=off  Pbase=100e6  Vbase=500e3  OutputType=Complex  PhasorSimulation=off  PSBequivalent=0
  Three-Phase Breaker : spsThreePhaseBreakerLib/Three-Phase Breaker  InitialState=closed  SwitchA=on  SwitchB=on  SwitchC=on  SwitchTimes="[1/60  5/60]"  External=on  BreakerResistance=0  SnubberResistance=1e4  SnubberCapacitance=inf  Measurements=None
  Three-Phase Source : spsThreePhaseSourceLib/Three-Phase Source  InternalConnection=Yg  VoltagePhases=off  Voltage=xs.sim.Vg*sqrt(3/2)  PhaseAngle=90  Voltage_phases=[25e3 25e3 25e3]/sqrt(3)  PhaseAngles_phases=[0 -120 +120]  Frequency=xs.sim.wg/(2*pi)  NonIdealSource=off  SpecifyImpedance=off  Resistance=0.8929  Inductance=16.58e-3  ShortCircuitLevel=100e6  BaseVoltage=25e3  XRratio=7  BusType=swing  Pref=10e3  Qref=0  Prefabc=[10e3, 10e3, 10e3]  Qrefabc=[0, 0, 0]  Qmin=-inf  Qmax=inf
  Two-Level Converter : spsTwoLevelConverterLib/Two-Level Converter  ModelType=Switching devices  Ron=1e-4  Rs=1e6  Cs=inf  Vforward=[0,0]  Ron_Diode=1e-2  Rs_Diode=1e4  Cs_Diode=inf  Vf_Diode=0  Rs_CurrentSource=inf  Ron_ACsource=1e-5
      settings: LibrarySourceBlock=sps_lib/Power Electronics/Two-Level Converter
  Zero-Order Hold : ZeroOrderHold  SampleTime=xs.model.Ts
  powergui : sps_lib/powergui  Priority=1  SimulationMode=Continuous  SampleTime=xs.model.Ts/5  frequency=60  Iterations=50  frequencyindice=0  Pbase=100e6  ErrMax=1e-4  UnitsV=kV  UnitsW=MW  buscounter=0  FunctionMessages=off  echomessages=off  EnableUseOfTLC=off  CurrentSourceSwitches=off  DisableSnubberDevices=off  DisableRonSwitches=off  DisableVfSwitches=off  DisplayEquations=off  AutomaticDiscreteSolvers=off  SolverType=Tustin/Backward Euler (TBE)  Interpol=off  ExternalGateDelay=off  methode=off  Ts=100  x0status=blocks  SPID=on  SwTol=0  HookPort=off  NonlinearTolerance=1e-4  nMaxIteration=100  ContinueOnMaxIteration=off  RestoreLinks=warning  ResistiveCurrentMeasurement=off  Frange=[0:2:500]  Ylog=off  Xlog=on  ShowGrid=off  save=off  variable=ZData  structure=0  ZoomFFT=off  StartTime=0.0  cycles=1  DisplayStyle=1  fundamental=60  FreqAxis=off  MaxFrequency=1000  frequencyindicesteady=1  RmsSteady=1  display=off
  xm : Outport
  tag scope: bkr=global, if_sims=global, ig_sims=global, vc_sims=global, vg_sims=global, vs_sims=global
  wires:
  Constant1/1 -> Two-Level Converter/2
  [vg_sims] -> Mux2/5, Scope2/5  "vg"
  [ig_sims] -> Mux2/3, Scope2/3  "ig"
  [if_sims] -> Mux2/1, Scope2/1  "if"
  [vs_sims] -> Mux2/2, Scope2/2  "vs"
  [vc] -> Mux2/4, Scope2/4  "vc"
  Three-Phase V-I Measurement/2 -> [if_sims]
  Three-Phase V-I Measurement2/1 -> [vg_sims]
  Three-Phase V-I Measurement2/2 -> [ig_sims]
  [if_sims] -> Mux1/1  "if"
  [vs_sims] -> Mux1/2  "vs"
  [ig_sims] -> Mux1/3  "ig"
  [vg_sims] -> Mux1/4  "vg"
  Three-Phase V-I Measurement/1 -> [vs_sims]
  Mux1/1 -> xm/1
  Three-Phase V-I Measurement1/1 -> [vc_sims]
  [vc_sims] -> Scope1/6, Scope2/6  "vc"
  Mux2/1 -> Zero-Order Hold/1
  Zero-Order Hold/1 -> Demux/1
  Demux/1 -> Scope1/1  "if"
  Demux/2 -> Scope1/2  "vs"
  Demux/3 -> Scope1/3  "ig"
  Demux/4 -> Scope1/4  "vc"
  Demux/5 -> Scope1/5  "vg"
  v_c/1 -> PWM/1(In1)
  PWM/1(Out1) -> Two-Level Converter/1
  Step/1 -> [bkr], Three-Phase Breaker/1
  connections:
  Two-Level Converter/RConn1 -- DC Voltage Source/RConn1
  Two-Level Converter/RConn2 -- DC Voltage Source/LConn1
  "Rf , Lf"/RConn1 -- Three-Phase V-I Measurement/LConn1
  "Rf , Lf"/RConn2 -- Three-Phase V-I Measurement/LConn2
  "Rf , Lf"/RConn3 -- Three-Phase V-I Measurement/LConn3
  Cf/LConn1 -- Three-Phase Breaker/LConn1 -- Three-Phase V-I Measurement/RConn1
  Cf/LConn2 -- Three-Phase V-I Measurement/RConn2 -- Three-Phase Breaker/LConn2
  Cf/LConn3 -- Three-Phase V-I Measurement/RConn3 -- Three-Phase Breaker/LConn3
  Three-Phase Source/RConn1 -- Three-Phase V-I Measurement2/RConn1
  Three-Phase Source/RConn2 -- Three-Phase V-I Measurement2/RConn2
  Three-Phase Source/RConn3 -- Three-Phase V-I Measurement2/RConn3
  Cf/RConn1 -- Cf/RConn2 -- Cf/RConn3
  Three-Phase V-I Measurement1/LConn2 -- Two-Level Converter/LConn2
  Two-Level Converter/LConn1 -- Three-Phase V-I Measurement1/LConn1
  Two-Level Converter/LConn3 -- Three-Phase V-I Measurement1/LConn3
  Three-Phase V-I Measurement1/RConn3 -- "Rf , Lf"/LConn3
  Three-Phase V-I Measurement1/RConn2 -- "Rf , Lf"/LConn2
  Three-Phase V-I Measurement1/RConn1 -- "Rf , Lf"/LConn1
  "Rg , Lg"/RConn1 -- Three-Phase V-I Measurement2/LConn1
  "Rg , Lg"/RConn2 -- Three-Phase V-I Measurement2/LConn2
  "Rg , Lg"/RConn3 -- Three-Phase V-I Measurement2/LConn3
  Three-Phase Breaker/RConn1 -- Ro/LConn1 -- "Rg , Lg"/LConn1
  Three-Phase Breaker/RConn2 -- Ro/LConn2 -- "Rg , Lg"/LConn2
  Three-Phase Breaker/RConn3 -- Ro/LConn3 -- "Rg , Lg"/LConn3
  Ro/RConn3 -- Ro/RConn1 -- Ro/RConn2

== system SIM_DNNs/Ref igdq1/Select_Ref ==
  In1 : Inport
  In2 : Inport  Port=2
  Product : Product
  Product1 : Product
  Ref_Rand : Constant  Value=1 - xs.sim.Ref_Rand
  Ref_Rand_neg : Constant  Value=xs.sim.Ref_Rand
  Sum1 : Sum  Inputs=|++
  r2k : Outport
  wires:
  Product1/1 -> Sum1/2
  Ref_Rand/1 -> Product/2
  In2/1 -> Product1/2
  Product/1 -> Sum1/1
  Ref_Rand_neg/1 -> Product1/1
  Sum1/1 -> r2k/1
  In1/1 -> Product/1

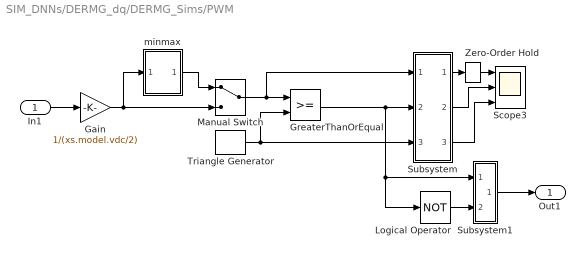
== system SIM_DNNs/DERMG_dq/DERMG_Sims/PWM ==
  In1 : Inport
  Gain : Gain  Gain=1/(xs.model.vdc/2)
  GreaterThanOrEqual : RelationalOperator  OutDataTypeStr=boolean  RndMeth=Simplest  InputSameDT=off
  Logical Operator : Logic  Operator=NOT  AllPortsSameDT=off  OutDataTypeStr=boolean
  Manual Switch : ManualSwitch
  Scope3 : Scope  NumInputPorts=3
  Subsystem : Subsystem
  Subsystem1 : Subsystem
  Triangle Generator : spsTriangleGeneratorLib/Triangle Generator  Freq=1/xs.model.Ts  Phase=0  Ts=0
  Zero-Order Hold : ZeroOrderHold  SampleTime=xs.model.Ts
  minmax : Subsystem
  Out1 : Outport
  wires:
  Triangle Generator/1 -> GreaterThanOrEqual/2, Subsystem/3(In3)
  In1/1 -> Gain/1
  Subsystem/2(Out2) -> Scope3/2
  Subsystem/3(Out3) -> Scope3/3
  GreaterThanOrEqual/1 -> Subsystem/2(In2), Subsystem1/1(In1), Logical Operator/1
  Logical Operator/1 -> Subsystem1/2(In2)
  Subsystem1/1(Out1) -> Out1/1
  Manual Switch/1 -> Subsystem/1(In1), GreaterThanOrEqual/1
  Gain/1 -> minmax/1(In1), Manual Switch/2
  minmax/1(Out1) -> Manual Switch/1
  Subsystem/1(Out1) -> Zero-Order Hold/1
  Zero-Order Hold/1 -> Scope3/1

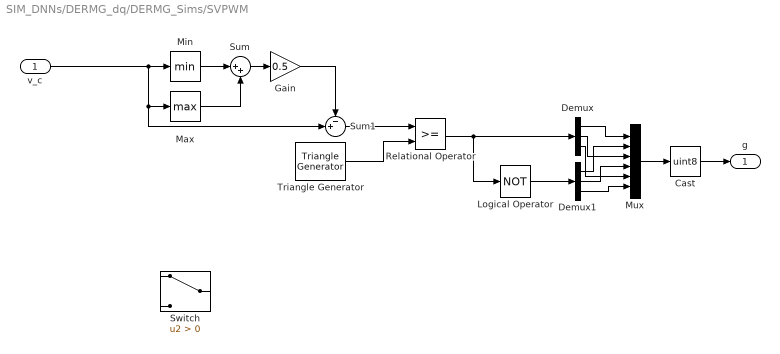
== system SIM_DNNs/DERMG_dq/DERMG_Sims/SVPWM ==
  v_c : Inport
  Cast : DataTypeConversion  OutDataTypeStr=uint8  SaturateOnIntegerOverflow=off  RndMeth=Floor
  Demux : Demux  Outputs=3
  Demux1 : Demux  Outputs=3
  Gain : Gain  Gain=0.5
  Logical Operator : Logic  Operator=NOT  AllPortsSameDT=off  OutDataTypeStr=boolean
  Max : MinMax  Function=max
  Min : MinMax
  Mux : Mux  Inputs=6
  Relational Operator : RelationalOperator  OutDataTypeStr=boolean  ZeroCross=off  RndMeth=Simplest  InputSameDT=off
  Sum : Sum  Inputs=|++
  Sum1 : Sum  Inputs=-+|
  Switch : Switch  Criteria=u2 > Threshold  SaturateOnIntegerOverflow=off  InputSameDT=off
  Triangle Generator : spsTriangleGeneratorLib/Triangle Generator  Freq=2/xs.model.Ts  Phase=0  Ts=0
  g : Outport
  wires:
  v_c/1 -> Max/1, Sum1/2, Min/1
  Sum1/1 -> Relational Operator/1
  Min/1 -> Sum/1
  Triangle Generator/1 -> Relational Operator/2
  Mux/1 -> Cast/1
  Max/1 -> Sum/2
  Demux/1 -> Mux/1
  Logical Operator/1 -> Demux1/1
  Sum/1 -> Gain/1
  Demux1/1 -> Mux/2
  Demux1/2 -> Mux/4
  Demux/3 -> Mux/5
  Relational Operator/1 -> Logical Operator/1, Demux/1
  Demux/2 -> Mux/3
  Demux1/3 -> Mux/6
  Cast/1 -> g/1
  Gain/1 -> Sum1/1

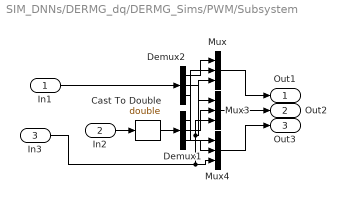
== system SIM_DNNs/DERMG_dq/DERMG_Sims/PWM/Subsystem ==
  In1 : Inport
  In2 : Inport  Port=2
  In3 : Inport  Port=3
  Cast To Double : DataTypeConversion  OutDataTypeStr=double  SaturateOnIntegerOverflow=off  RndMeth=Floor
  Demux1 : Demux  Outputs=3
  Demux2 : Demux  Outputs=3
  Mux : Mux  Inputs=3
  Mux3 : Mux  Inputs=3
  Mux4 : Mux  Inputs=3
  Out1 : Outport
  Out2 : Outport  Port=2
  Out3 : Outport  Port=3
  wires:
  Demux2/2 -> Mux3/1
  In2/1 -> Cast To Double/1
  In3/1 -> Mux3/3, Mux/3, Mux4/3
  Cast To Double/1 -> Demux1/1
  Demux2/3 -> Mux4/1
  Demux1/1 -> Mux/2
  Demux1/3 -> Mux4/2
  Demux2/1 -> Mux/1
  Demux1/2 -> Mux3/2
  Mux/1 -> Out1/1
  Mux3/1 -> Out2/1
  Mux4/1 -> Out3/1
  In1/1 -> Demux2/1

== system SIM_DNNs/DERMG_dq/DERMG_Sims/PWM/Subsystem1 ==
  In1 : Inport
  In2 : Inport  Port=2
  Cast To Double1 : DataTypeConversion  OutDataTypeStr=double  SaturateOnIntegerOverflow=off  RndMeth=Floor
  Demux3 : Demux  Outputs=3
  Demux4 : Demux  Outputs=3
  Mux5 : Mux  Inputs=6
  Out1 : Outport
  wires:
  Mux5/1 -> Cast To Double1/1
  Demux3/3 -> Mux5/5
  Demux3/2 -> Mux5/3
  Demux4/1 -> Mux5/2
  Demux4/2 -> Mux5/4
  Demux3/1 -> Mux5/1
  Demux4/3 -> Mux5/6
  In2/1 -> Demux4/1
  Cast To Double1/1 -> Out1/1
  In1/1 -> Demux3/1

== system SIM_DNNs/DERMG_dq/DERMG_Sims/PWM/minmax ==
  In1 : Inport
  Gain1 : Gain  Gain=0.5
  Max : MinMax  Function=max
  Min : MinMax
  Sum : Sum  Inputs=|++
  Sum1 : Sum  Inputs=-+|
  Out1 : Outport
  wires:
  In1/1 -> Max/1, Min/1, Sum1/2
  Sum/1 -> Gain1/1
  Gain1/1 -> Sum1/1
  Max/1 -> Sum/2
  Min/1 -> Sum/1
  Sum1/1 -> Out1/1

== matlab function SIM_DNNs/DERMG_dq/MATLAB Function2 ==
  data: wt input; s_dq output size=2; s_abc input size=3
function s_dq = abc2dq(wt,s_abc)

% ABC to DQ0 transformation
% s_abc = [a;b;c]
% s_dq0 = [d;q;0]

% Clarke transformation matrix, depends on the electrical angle
T = (2/3)*[cos(wt) cos(wt-2*pi/3) cos(wt+2*pi/3);...
    -sin(wt) -sin(wt-2*pi/3) -sin(wt+2*pi/3);...
    0.5 0.5 0.5];

% DQ0 transformation (only D and Q components are needed)
s_dq0 = T*s_abc;
s_dq = s_dq0(1:2);

end

== matlab function SIM_DNNs/DERMG_dq/MATLAB Function3 ==
  data: wt input; s_dq output size=2; s_abc input size=3
function s_dq = abc2dq(wt,s_abc)

% ABC to DQ0 transformation
% s_abc = [a;b;c]
% s_dq0 = [d;q;0]

% Clarke transformation matrix, depends on the electrical angle
T = (2/3)*[cos(wt) cos(wt-2*pi/3) cos(wt+2*pi/3);...
    -sin(wt) -sin(wt-2*pi/3) -sin(wt+2*pi/3);...
    0.5 0.5 0.5];

% DQ0 transformation (only D and Q components are needed)
s_dq0 = T*s_abc;
s_dq = s_dq0(1:2);

end

== matlab function SIM_DNNs/DERMG_dq/MATLAB Function4 ==
  data: wt input; s_abc output; s_dq input
function s_abc = dq2abc(wt,s_dq)

% DQ0 to ABC transformation
% s_dq0 = [d;q;0]
% s_abc = [a;b;c]

% Inverse Clarke transformation matrix, depends on the electrical angle
Tinv = [cos(wt) -sin(wt) 1;...
    cos(wt-2*pi/3) -sin(wt-2*pi/3) 1;...
    cos(wt+2*pi/3) -sin(wt+2*pi/3) 1];

s_dq0 = [s_dq;0];
s_abc = Tinv*s_dq0;

end

== matlab function SIM_DNNs/DNN Control/MATLAB Function1 ==
  data: xk1 input size=4; theta_c input size=1; uk1_proj output size=2; dk1 input size=2; rk1 input size=1; dik input size=2; xproj1 parameter; xtime output size=1; parsDNN1 parameter; mins_max1 parameter; eval_net_func1 parameter; xmpc1 parameter; use_net1 parameter
function [uk1_proj, xtime] = DNN1(xk1, theta_c, dk1, rk1, dik,xproj1, parsDNN1, mins_max1, eval_net_func1, xmpc1, use_net1)

tStart = tic;
persistent F_
if(use_net1)
    X1 = [xk1; dk1; rk1; cos(theta_c); sin(theta_c)];
    if isempty(F_)
        F_ = fimath('OverflowAction', 'Saturate', ... 
           'RoundingMethod', 'Convergent', ...
           'ProductMode', 'SpecifyPrecision', ...
           'ProductWordLength', parsDNN1.wordLength, ...
           'ProductFractionLength', parsDNN1.fracLength, ...
           'SumMode', 'SpecifyPrecision', ...
           'SumWordLength', parsDNN1.wordLength, ...
           'SumFractionLength', parsDNN1.fracLength);
    end
    %Normalizar
    x_norm = (X1 - mins_max1.in_min) ./ (mins_max1.in_max - mins_max1.in_min);
    %Evaluar
    eval_net_func_char = char(eval_net_func1);
    uk_net1 = double(zeros(size(mins_max1.out_max)));
    uk_net1 = feval(eval_net_func_char,x_norm, parsDNN1, F_);
    %Desnormalizar
    uk_net1 = (mins_max1.out_max - mins_max1.out_min).*uk_net1 + mins_max1.out_min;
    % Output Saturation/Projection
    %uk1_proj = uk_net1 - dik;
    uk1_proj = Project1_f(xk1, uk_net1 - dik, dk1, theta_c, xproj1);
    %uk1_proj= uk_net1;
    % %uk1_proj = min(max(uk1_proj, mins_max1.out_min), mins_max1.out_max);
else
    uk1_proj = MPC1_f(xk1,dk1,[rk1;0],dik,theta_c,xmpc1);
end
xtime = toc(tStart);

end

== matlab function SIM_DNNs/DERMG_dq/DERMG_EQabc/MATLAB Function ==
  data: i_f input; di_f output; v_s input; i_g input; v_c input; v_g input; bkr input; dv_s output; di_g output; xs parameter
function [di_f,dv_s,di_g] = DERMG_SYSEQabc(i_f,v_s,i_g,v_c,v_g,bkr,xs)


[di_f,dv_s,di_g] = DERMG_SYSEQabc_f(i_f,v_s,i_g,v_c,v_g,bkr,xs);


end

== matlab function SIM_DNNs/DERMG_dq/MATLAB Function1 ==
  data: wt input; s_dq output size=2; s_abc input size=3
function s_dq = abc2dq(wt,s_abc)

% ABC to DQ0 transformation
% s_abc = [a;b;c]
% s_dq0 = [d;q;0]

% Clarke transformation matrix, depends on the electrical angle
T = (2/3)*[cos(wt) cos(wt-2*pi/3) cos(wt+2*pi/3);...
    -sin(wt) -sin(wt-2*pi/3) -sin(wt+2*pi/3);...
    0.5 0.5 0.5];

% DQ0 transformation (only D and Q components are needed)
s_dq0 = T*s_abc;
s_dq = s_dq0(1:2);

end

== matlab function SIM_DNNs/DERMG_dq/MATLAB Function5 ==
  data: wt input; s_dq output size=2; s_abc input size=3
function s_dq = abc2dq(wt,s_abc)

% ABC to DQ0 transformation
% s_abc = [a;b;c]
% s_dq0 = [d;q;0]

% Clarke transformation matrix, depends on the electrical angle
T = (2/3)*[cos(wt) cos(wt-2*pi/3) cos(wt+2*pi/3);...
    -sin(wt) -sin(wt-2*pi/3) -sin(wt+2*pi/3);...
    0.5 0.5 0.5];

% DQ0 transformation (only D and Q components are needed)
s_dq0 = T*s_abc;
s_dq = s_dq0(1:2);

end

== matlab function SIM_DNNs/DERMG_dq/MATLAB Function6 ==
  data: s_ab output size=2; s_abc input size=3
function s_ab = abc2alphabeta(s_abc)

T = [[2/3, -1/3, -1/3]; [0, 1/sqrt(3), -1/sqrt(3)]];

s_ab = T*s_abc;

end

== matlab function SIM_DNNs/DNN Control/MATLAB Function ==
  data: xk2 input size=3; uk_net2 output size=2; dk2 input size=2; rk2 input size=2; xsat2 parameter; xtime output size=1; parsDNN2 parameter; mins_max2 parameter; eval_net_func2 parameter; xmpc2 parameter; use_net2 parameter
function [uk_net2, xtime] = DNN2(xk2, dk2, rk2, xsat2, parsDNN2, mins_max2, eval_net_func2, xmpc2, use_net2)

    tStart = tic;
    persistent F_
    rk2_sat = SAT_f(rk2,xsat2);
    if(use_net2)
        if isempty(F_)
            F_ = fimath('OverflowAction', 'Saturate', ... 
               'RoundingMethod', 'Convergent', ...
               'ProductMode', 'SpecifyPrecision', ...
               'ProductWordLength', parsDNN2.wordLength, ...
               'ProductFractionLength', parsDNN2.fracLength, ...
               'SumMode', 'SpecifyPrecision', ...
               'SumWordLength', parsDNN2.wordLength, ...
               'SumFractionLength', parsDNN2.fracLength);
        end
        X2 = [xk2; dk2; rk2_sat];
        %Normalizar
        x_norm = (X2 - mins_max2.in_min) ./ (mins_max2.in_max - mins_max2.in_min);
        %Evaluar
        eval_net_func_char = char(eval_net_func2);
        uk_net2 = double(zeros(size(mins_max2.out_max)));
        uk_net2 = feval(eval_net_func_char,x_norm, parsDNN2, F_);
        %Desnormalizar
        uk_net2 = (mins_max2.out_max - mins_max2.out_min).*uk_net2 + mins_max2.out_min;
        %uk_net2 = min(max(uk_net2, mins_max2.out_min), mins_max2.out_max);
    else
        [uk_net2,~] = MPC2_f(xk2,dk2,rk2_sat,xmpc2);
    end
    xtime = toc(tStart);

end
